simulink model "sim_bounded_varbounded_noise"  (R2018b)
settings: Solver=VariableStepAuto  StartTime=0.0  StopTime=10.0  RelTol=1e-3
undefined symbols (not defined in the file or in its folder): DiscIntNeverNeededParam, dp_lim, np, p_lim, p_nom
libraries: dspsrcs4 x2
settings Model: Creator=ppolcz  LastModifiedBy=ppolcz

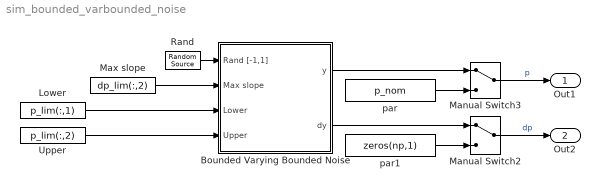
== system sim_bounded_varbounded_noise ==
  Bounded Varying Bounded Noise : Subsystem
  Lower : Constant  Value=p_lim(:,1)
  Manual Switch2 : ManualSwitch
  Manual Switch3 : ManualSwitch
  Max slope : Constant  Value=dp_lim(:,2)
  Rand : dspsrcs4/Random Source  SrcType=Gaussian  NormMethod=Ziggurat  CltLength=12  MinVal=-1  MaxVal=1  MeanVal=gaussrand_mean  VarVal=gaussrand_var  RepMode=Not repeatable  rawSeed=1  IsInherit=off  SampMode=Discrete  SampTime=0.1  SampFrame=1  DataType=Double  OutComplex=Real  OutputFrames=off
  Upper : Constant  Value=p_lim(:,2)
  par : Constant  Value=p_nom
  par1 : Constant  Value=zeros(np,1)
  Out1 : Outport
  Out2 : Outport  Port=2
  wires:
  Bounded Varying Bounded Noise/2(dy) -> Manual Switch2/1
  Upper/1 -> Bounded Varying Bounded Noise/4(Upper)
  Manual Switch2/1 -> Out2/1  "dp"
  par1/1 -> Manual Switch2/2
  Bounded Varying Bounded Noise/1(y) -> Manual Switch3/1
  Manual Switch3/1 -> Out1/1  "p"
  Rand/1 -> Bounded Varying Bounded Noise/1(Rand [-1,1])
  Max slope/1 -> Bounded Varying Bounded Noise/2(Max slope)
  par/1 -> Manual Switch3/2
  Lower/1 -> Bounded Varying Bounded Noise/3(Lower)

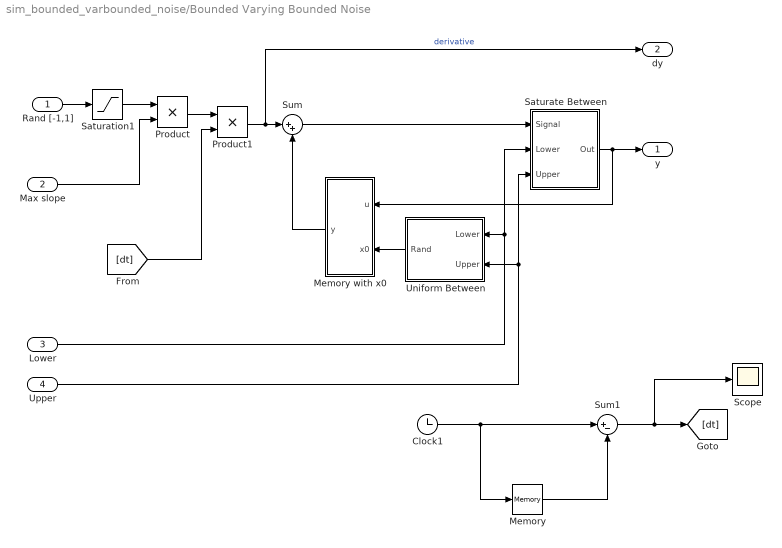
== system sim_bounded_varbounded_noise/Bounded Varying Bounded Noise ==
  Rand [-1,1] : Inport
  Max slope : Inport  Port=2
  Lower : Inport  Port=3
  Upper : Inport  Port=4
  Clock1 : Clock
  Memory : Memory
  Memory with x0 : Subsystem
  Product : Product
  Product1 : Product
  Saturate Between : Subsystem
  Saturation1 : Saturate  UpperLimit=1  LowerLimit=-1
  Scope : Scope
  Sum : Sum  Inputs=|++
  Sum1 : Sum  Inputs=|+-
  Uniform Between : Subsystem
  y : Outport
  dy : Outport  Port=2
  wires:
  Saturation1/1 -> Product/1
  Rand [-1,1]/1 -> Saturation1/1
  Sum/1 -> Saturate Between/1(Signal)
  Memory with x0/1(y) -> Sum/2
  Uniform Between/1(Rand) -> Memory with x0/2(x0)
  Upper/1 -> Uniform Between/2(Upper), Saturate Between/3(Upper)
  Lower/1 -> Uniform Between/1(Lower), Saturate Between/2(Lower)
  Saturate Between/1(Out) -> Memory with x0/1(u), y/1
  Max slope/1 -> Product/2
  Clock1/1 -> Memory/1, Sum1/1
  Sum1/1 -> [dt], Scope/1
  Memory/1 -> Sum1/2
  Product1/1 -> dy/1, Sum/1  "derivative"
  Product/1 -> Product1/1
  [dt] -> Product1/2

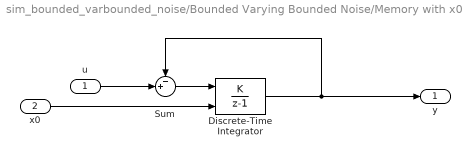
== system sim_bounded_varbounded_noise/Bounded Varying Bounded Noise/Memory with x0 ==
  u : Inport
  x0 : Inport  Port=2
  Discrete-Time Integrator : DiscreteIntegrator  IntegratorMethod=Accumulation: Forward Euler  InitialConditionSource=external  SampleTime=-1  ICPrevOutput=DiscIntNeverNeededParam  ICPrevScaledInput=DiscIntNeverNeededParam
  Sum : Sum  Inputs=-+|
  y : Outport
  wires:
  u/1 -> Sum/2
  Sum/1 -> Discrete-Time Integrator/1
  x0/1 -> Discrete-Time Integrator/2
  Discrete-Time Integrator/1 -> y/1, Sum/1

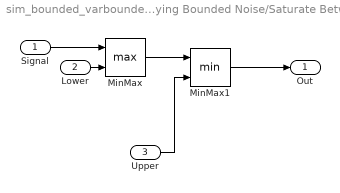
== system sim_bounded_varbounded_noise/Bounded Varying Bounded Noise/Saturate Between ==
  Signal : Inport
  Lower : Inport  Port=2
  Upper : Inport  Port=3
  MinMax : MinMax  Function=max  Inputs=2
  MinMax1 : MinMax  Inputs=2
  Out : Outport
  wires:
  MinMax/1 -> MinMax1/1
  Lower/1 -> MinMax/2
  Upper/1 -> MinMax1/2
  MinMax1/1 -> Out/1
  Signal/1 -> MinMax/1

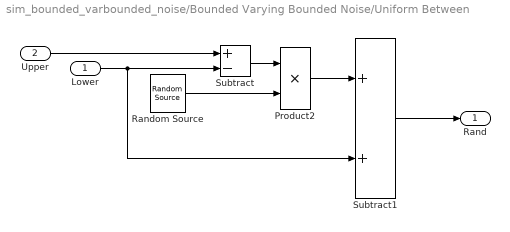
== system sim_bounded_varbounded_noise/Bounded Varying Bounded Noise/Uniform Between ==
  Lower : Inport
  Upper : Inport  Port=2
  Product2 : Product
  "Random Source " : dspsrcs4/Random Source  SrcType=Uniform  NormMethod=Ziggurat  CltLength=12  MinVal=rand2_mean  MaxVal=rand2_var  MeanVal=0  VarVal=1  RepMode=Not repeatable  rawSeed=1  IsInherit=off  SampMode=Discrete  SampTime=0.1  SampFrame=1  DataType=Double  OutComplex=Real  OutputFrames=off
  Subtract : Sum  Inputs=+-
  Subtract1 : Sum
  Rand : Outport
  wires:
  "Random Source "/1 -> Product2/2
  Product2/1 -> Subtract1/1
  Upper/1 -> Subtract/1
  Subtract/1 -> Product2/1
  Lower/1 -> Subtract1/2, Subtract/2
  Subtract1/1 -> Rand/1
